simulink model "DLC_2a"  (R2023a)
settings: Solver=ode4  StartTime=0.0  StopTime=40  FixedStep=0.005  RelTol=1e-3
InitFcn:
  | DLC2
values from neighbouring files (symbols this model uses):
  K_scheduled = zeros(length(V_op), 2)    [CAL3.m]    (also in CUB.m; DLC2.m; MUS.m; OHZ.m)
  V_op = 5:5:85    [CAL3.m]    (also in CUB.m; DLC2.m; MUS.m; OHZ.m)
  X_track = [linspace(0, runway_length, 200)'; runway_length + R_track * cos(theta_circ(2:end))]    [CAL3.m]    (also in CUB.m = [0; 5000]; DLC2.m = 0:0.1:total_track_length; MUS.m = [0; 2000]; OHZ.m = [0; 2000])
  Y_track = [zeros(200, 1); R_track + R_track * sin(theta_circ(2:end))]    [CAL3.m]    (also in CUB.m = [0; 0]; DLC2.m = zeros(size(X_track)); MUS.m = [0; 0]; OHZ.m = [0; 0])
undefined symbols (not defined in the file or in its folder): planner_params, track_params, veh_params
libraries: simulink x2, slpidlib x2
(part 3 of 3)

== matlab function DLC_2a/Track & Environment references/MATLAB Function ==
  settings: updateMethod=DISCRETE
  data: X_veh input; v_ref output; Y_veh input; psi_veh input; vx input; kappa_ref output; psi_ref output; delta_cmd output; current_idx_out output; planner_params parameter; veh_params parameter; track_params parameter; sim_time input; recovery_active output; prev_idx_in input
function [v_ref, kappa_ref, psi_ref, delta_cmd, current_idx_out, recovery_active] = dlc_pure_pursuit_planner(X_veh, Y_veh, psi_veh, vx, planner_params, veh_params, track_params, sim_time, prev_idx_in)
    % =========================================================================
    % ISO DLC PURE PURSUIT PLANNER (User Recovery Logic Version)
    % =========================================================================
    
    % -------------------------------------------------------------------------
    % 0. UNPACK PARAMETERS TO MATCH USER VARIABLES
    % -------------------------------------------------------------------------
    X_curr = X_veh(1); 
    Y_curr = Y_veh(1); 
    psi_curr = psi_veh(1); 
    vx_curr = vx(1);
    
    L = veh_params.L;
    
    X_track = track_params.X;
    Y_track = track_params.Y;
    s_track = track_params.s;
    V_profile = track_params.vx;
    kappa_track = track_params.kappa;
    psi_track = track_params.psi;

    % -------------------------------------------------------------------------
    % 1. USER'S UNTOUCHED CORE LOGIC
    % -------------------------------------------------------------------------
    persistent recovery_start_time tube_exceeded
    if isempty(recovery_start_time); recovery_start_time = -10; end
    if isempty(tube_exceeded); tube_exceeded = 0; end
    
    dist_sq = (X_track - X_curr).^2 + (Y_track - Y_curr).^2;
    [min_dist_sq, min_idx] = min(dist_sq);
    e_ct = sqrt(min_dist_sq); 
    
    % Map to the required interface output
    current_idx_out = min_idx; 
    
    tube_limit = 10.0; 
    if e_ct > tube_limit && tube_exceeded == 0
        tube_exceeded = 1;
        recovery_start_time = sim_time;
    end
    
    if sim_time - recovery_start_time < 1.0
        recovery_active = 1;
        v_ref = 0.0; 
        delta_cmd = 0.0; 
        kappa_ref = 0.0;
        psi_ref = psi_track(min_idx);
        return; 
    else
        recovery_active = 0;
        if e_ct < 2.0; tube_exceeded = 0; end 
    end
    
    vx_safe = max(vx_curr, 2.0); 
    Ld = max(15.0, 1.2 * vx_safe); 
    
    idx_target = min_idx;
    while idx_target < length(s_track) && (s_track(idx_target) - s_track(min_idx)) < Ld
        idx_target = idx_target + 1;
    end
    
    X_target = X_track(idx_target); 
    Y_target = Y_track(idx_target);
    
    alpha = atan2(Y_target - Y_curr, X_target - X_curr) - psi_curr;
    alpha = mod(alpha + pi, 2*pi) - pi;
    
    delta_cmd = atan2(2 * L * sin(alpha), Ld);
    kappa_cmd = (2 * sin(alpha)) / Ld;
    
    % =====================================================================
    % --- CONSTANT SPEED OVERRIDE FOR DLC TEST ---
    % =====================================================================
    % The planner will no longer reduce speed for sharp corners. 
    % It strictly commands the profile speed defined in the startup script.
    v_ref = V_profile(min_idx);
    % =====================================================================
    
    kappa_ref = kappa_cmd;
    psi_ref = psi_track(min_idx);
end
